simulink model "FIR_fixed"  (R2017a)
settings: Solver=VariableStepAuto  StartTime=0.0  StopTime=10.0  RelTol=1e-3
settings Model: Creator=Arthur  LastModifiedBy=Arthur

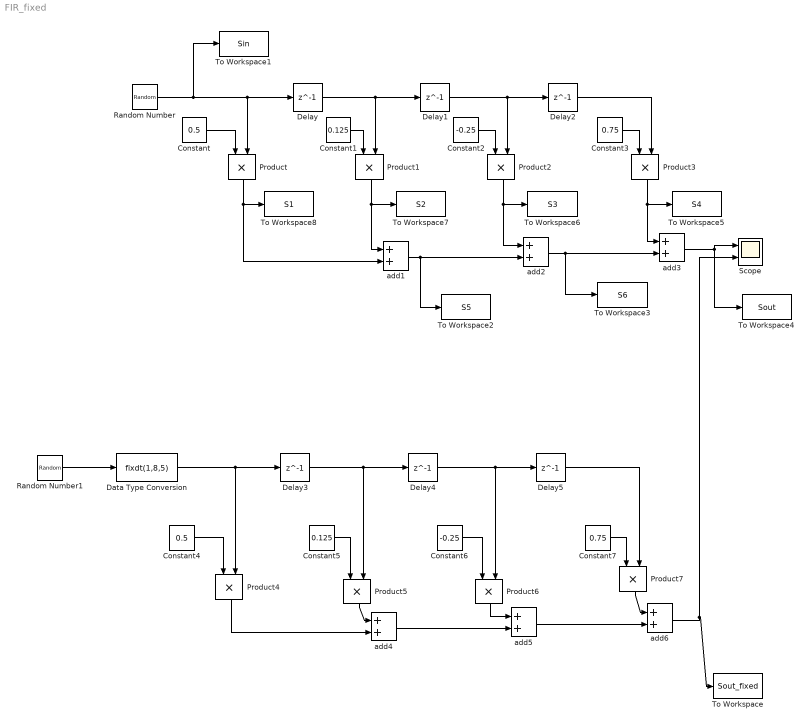
== system FIR_fixed ==
  Constant : Constant  Value=0.5
  Constant1 : Constant  Value=0.125
  Constant2 : Constant  Value=-0.25
  Constant3 : Constant  Value=0.75
  Constant4 : Constant  Value=0.5  OutDataTypeStr=fixdt(0,1,1)
  Constant5 : Constant  Value=0.125  OutDataTypeStr=fixdt(0,3,3)
  Constant6 : Constant  Value=-0.25  OutDataTypeStr=fixdt(1,3,2)
  Constant7 : Constant  Value=0.75  OutDataTypeStr=fixdt(0,2,2)
  Data Type Conversion : DataTypeConversion  OutDataTypeStr=fixdt(1,8,5)
  Delay{,1..5} (6 alike) : Delay  DelayLength=1
  Product{,1..3} (4 alike) : Product
  Product4 : Product  OutDataTypeStr=fixdt(1,8,6)
  Product5 : Product  OutDataTypeStr=fixdt(1,8,7)
  Product6 : Product  OutDataTypeStr=fixdt(1,8,7)
  Product7 : Product  OutDataTypeStr=fixdt(1,8,6)
  Random Number : RandomNumber  SampleTime=0.1
  Random Number1 : RandomNumber  SampleTime=0.1
  Scope : Scope  NumInputPorts=2
  To Workspace : ToWorkspace  VariableName=Sout_fixed  SampleTime=-1
  To Workspace1 : ToWorkspace  VariableName=Sin  SampleTime=-1
  To Workspace2 : ToWorkspace  VariableName=S5  SampleTime=-1
  To Workspace3 : ToWorkspace  VariableName=S6  SampleTime=-1
  To Workspace4 : ToWorkspace  VariableName=Sout  SampleTime=-1
  To Workspace5 : ToWorkspace  VariableName=S4  SampleTime=-1
  To Workspace6 : ToWorkspace  VariableName=S3  SampleTime=-1
  To Workspace7 : ToWorkspace  VariableName=S2  SampleTime=-1
  To Workspace8 : ToWorkspace  VariableName=S1  SampleTime=-1
  add1 : Sum
  add2 : Sum
  add3 : Sum
  add4 : Sum  OutDataTypeStr=fixdt(1,8,6)
  add5 : Sum  OutDataTypeStr=fixdt(1,8,6)
  add6 : Sum  OutDataTypeStr=fixdt(1,8,5)
  wires:
  Product1/1 -> To Workspace7/1, add1/1
  add1/1 -> To Workspace2/1, add2/2
  Product/1 -> To Workspace8/1, add1/2
  Constant/1 -> Product/1
  add3/1 -> To Workspace4/1, Scope/1
  Constant3/1 -> Product3/1
  Constant2/1 -> Product2/1
  Delay2/1 -> Product3/2
  Constant1/1 -> Product1/1
  Product2/1 -> To Workspace6/1, add2/1
  add2/1 -> To Workspace3/1, add3/2
  Product3/1 -> To Workspace5/1, add3/1
  Delay/1 -> Product1/2, Delay1/1
  Delay1/1 -> Product2/2, Delay2/1
  Random Number/1 -> To Workspace1/1, Product/2, Delay/1
  Random Number1/1 -> Data Type Conversion/1
  Product6/1 -> add5/1
  Constant5/1 -> Product5/1
  Delay5/1 -> Product7/2
  Constant6/1 -> Product6/1
  add4/1 -> add5/2
  Product4/1 -> add4/2
  Product5/1 -> add4/1
  add5/1 -> add6/2
  Constant4/1 -> Product4/1
  Delay3/1 -> Product5/2, Delay4/1
  Constant7/1 -> Product7/1
  Delay4/1 -> Product6/2, Delay5/1
  Product7/1 -> add6/1
  Data Type Conversion/1 -> Product4/2, Delay3/1
  add6/1 -> To Workspace/1, Scope/2
